simulink model "pd_path_sg"  (R2013b)
settings: Solver=ode45  StartTime=0.0  StopTime=10  RelTol=1e-3
undefined symbols (not defined in the file or in its folder): A, A2, B, C, D, EVAL, i, output_samp_bcoef, PCIN, reg_pk_lim, reg_plim, reg_scale, reg_sr_lim, reg_staclr, reg_txgain, THIS_DATE, W, X, Z
undefined symbols (not defined in the file): lut_address, lut_address_s5, reg_dltap
libraries: xbsIndex_r4 x3819, lut_ram_vhdl x32
(part 5 of 31)

== system pd_path_sg/B_dispatch/vdelay6 ==
  dn : Inport
  x : Inport  Port=2
  ab : Inport  Port=3
  Mux : Mux  Inputs=2
  Reinterpret : xbsIndex_r4/Reinterpret  force_arith_type=on  arith_type="Signed  (2's comp)"  force_bin_pt=on  bin_pt=0  block_type=reinterpret
  Reinterpret1 : xbsIndex_r4/Reinterpret  force_arith_type=on  arith_type="Signed  (2's comp)"  force_bin_pt=on  bin_pt=0  block_type=reinterpret
  Slice : xbsIndex_r4/Slice  nbits=6  boolean_output=off  mode=Lower Bit Location + Width  bit1=0  base1=MSB of Input  bit0=0  base0=LSB of Input  dbl_ovrd=off  block_type=slice
  Slice1 : xbsIndex_r4/Slice  nbits=6  boolean_output=off  mode=Lower Bit Location + Width  bit1=0  base1=MSB of Input  bit0=8  base0=LSB of Input  dbl_ovrd=off  block_type=slice
  Slice2 : xbsIndex_r4/Slice  nbits=16  boolean_output=off  mode=Lower Bit Location + Width  bit1=0  base1=MSB of Input  bit0=16  base0=LSB of Input  dbl_ovrd=off  block_type=slice
  Slice3 : xbsIndex_r4/Slice  nbits=16  boolean_output=off  mode=Lower Bit Location + Width  bit1=0  base1=MSB of Input  bit0=0  base0=LSB of Input  dbl_ovrd=off  block_type=slice
  Slice4 : xbsIndex_r4/Slice  nbits=10  boolean_output=off  mode=Lower Bit Location + Width  bit1=0  base1=MSB of Input  bit0=10  base0=LSB of Input  dbl_ovrd=off  block_type=slice
  Slice5 : xbsIndex_r4/Slice  nbits=10  boolean_output=off  mode=Lower Bit Location + Width  bit1=0  base1=MSB of Input  bit0=0  base0=LSB of Input  dbl_ovrd=off  block_type=slice
  asr0 : xbsIndex_r4/Addressable Shift Register  infer_latency=on  depth=64  initVector=[0]  en=off  use_behavioral_HDL=off  Optimization=Resource  dbl_ovrd=off  block_type=addrsr
      settings: infoedit="Delay of configurable length.  Any element in the delay line can be addressed and driven onto the output port.<br><br>Hardware notes: Generates fast, compact FIFO-style shift registers or delay lines using SRL16/SRL32 mode of the slice LUTs"
  asr1 : xbsIndex_r4/Addressable Shift Register  infer_latency=on  depth=64  initVector=[0]  en=off  use_behavioral_HDL=off  Optimization=Resource  dbl_ovrd=off  block_type=addrsr
      settings: infoedit="Delay of configurable length.  Any element in the delay line can be addressed and driven onto the output port.<br><br>Hardware notes: Generates fast, compact FIFO-style shift registers or delay lines using SRL16/SRL32 mode of the slice LUTs"
  regsp : xbsIndex_r4/Delay  rst=off  infoeditControl=Selection of Reset will increase slice count due to use of real FFs and instead of SRLs  en=off  latency=1  reg_retiming=off  dbl_ovrd=off  block_type=delay
      settings: infoedit=Hardware notes: A delay line is a chain, each link of which is an SRL16 or SRL32 followed by a flip-flop.
  regsp1 : xbsIndex_r4/Delay  rst=off  infoeditControl=Selection of Reset will increase slice count due to use of real FFs and instead of SRLs  en=off  latency=1  reg_retiming=off  dbl_ovrd=off  block_type=delay
      settings: infoedit=Hardware notes: A delay line is a chain, each link of which is an SRL16 or SRL32 followed by a flip-flop.
  y : Outport
  ar : Outport  Port=2
  br : Outport  Port=3
  wires:
  Reinterpret1/1 -> Mux/2
  Reinterpret/1 -> Mux/1
  Mux/1 -> y/1
  Slice3/1 -> Reinterpret1/1
  Slice2/1 -> Reinterpret/1
  dn/1 -> Slice/1, Slice1/1
  Slice5/1 -> br/1
  Slice4/1 -> ar/1
  asr1/1 -> regsp1/1
  asr0/1 -> regsp/1
  x/1 -> asr0/1
  Slice/1 -> asr0/2
  ab/1 -> asr1/1
  Slice1/1 -> asr1/2
  regsp/1 -> Slice2/1, Slice3/1
  regsp1/1 -> Slice5/1, Slice4/1

== system pd_path_sg/B_lut_store/one_lut0 ==
  chn_seq : Inport
  active0 : Inport  Port=2
  active1 : Inport  Port=3
  a : Inport  Port=4
  b : Inport  Port=5
  per_wr : Inport  Port=6
  B : Subsystem
  Bf : Subsystem
  Bp1 : Subsystem
  Bus Selector : BusSelector  OutputSignals=addr,din,we,chnsel,bandsel ,active,per_clk
  Bus Selector1 : BusSelector  OutputSignals=addr,din,we,chnsel,bandsel ,active,per_clk
  Constant : xbsIndex_r4/Constant  const=band_sel  gui_display_data_type=Fixed-point  arith_type=Unsigned  n_bits=1  bin_pt=0  preci_type=Single  exp_width=8  frac_width=24  explicit_period=off  period=1  equ=P=C  opselect=C  inp2=PCIN>>17  opr=+  inp1=P  carry=CIN  dbl_ovrd=off  block_type=constant
  Constant1 : xbsIndex_r4/Constant  const=lut_addr  gui_display_data_type=Fixed-point  arith_type=Unsigned  n_bits=4  bin_pt=0  preci_type=Single  exp_width=8  frac_width=24  explicit_period=off  period=1  equ=P=C  opselect=C  inp2=PCIN>>17  opr=+  inp1=P  carry=CIN  dbl_ovrd=off  block_type=constant
  Constant2 : xbsIndex_r4/Constant  const=0  gui_display_data_type=Fixed-point  arith_type=Unsigned  n_bits=1  bin_pt=0  preci_type=Single  exp_width=8  frac_width=24  explicit_period=off  period=1  equ=P=C  opselect=C  inp2=PCIN>>17  opr=+  inp1=P  carry=CIN  dbl_ovrd=off  block_type=constant
  Constant3 : xbsIndex_r4/Constant  const=band_sel  gui_display_data_type=Fixed-point  arith_type=Unsigned  n_bits=1  bin_pt=0  preci_type=Single  exp_width=8  frac_width=24  explicit_period=off  period=1  equ=P=C  opselect=C  inp2=PCIN>>17  opr=+  inp1=P  carry=CIN  dbl_ovrd=off  block_type=constant
  Constant4 : xbsIndex_r4/Constant  const=lut_addr  gui_display_data_type=Fixed-point  arith_type=Unsigned  n_bits=4  bin_pt=0  preci_type=Single  exp_width=8  frac_width=24  explicit_period=off  period=1  equ=P=C  opselect=C  inp2=PCIN>>17  opr=+  inp1=P  carry=CIN  dbl_ovrd=off  block_type=constant
  Constant5 : xbsIndex_r4/Constant  const=1  gui_display_data_type=Fixed-point  arith_type=Unsigned  n_bits=1  bin_pt=0  preci_type=Single  exp_width=8  frac_width=24  explicit_period=off  period=1  equ=P=C  opselect=C  inp2=PCIN>>17  opr=+  inp1=P  carry=CIN  dbl_ovrd=off  block_type=constant
  Convert : xbsIndex_r4/Convert  gui_display_data_type=Fixed-point  arith_type=Unsigned  n_bits=8  bin_pt=0  float_type=Single  exp_bits=8  fraction_bits=24  quantization=Truncate  overflow=Wrap  en=off  latency=0  pipeline=off  dbl_ovrd=off  block_type=convert
  Delay : xbsIndex_r4/Delay  rst=off  infoeditControl=Selection of Reset will increase slice count due to use of real FFs and instead of SRLs  en=off  latency=4  reg_retiming=off  dbl_ovrd=off  block_type=delay
      settings: infoedit=Hardware notes: A delay line is a chain, each link of which is an SRL16 or SRL32 followed by a flip-flop.
  Delay1 : xbsIndex_r4/Delay  rst=off  infoeditControl=Selection of Reset will increase slice count due to use of real FFs and instead of SRLs  en=off  latency=4  reg_retiming=off  dbl_ovrd=off  block_type=delay
      settings: infoedit=Hardware notes: A delay line is a chain, each link of which is an SRL16 or SRL32 followed by a flip-flop.
  Delay2 : xbsIndex_r4/Delay  rst=off  infoeditControl=Selection of Reset will increase slice count due to use of real FFs and instead of SRLs  en=off  latency=8  reg_retiming=off  dbl_ovrd=off  block_type=delay
      settings: infoedit=Hardware notes: A delay line is a chain, each link of which is an SRL16 or SRL32 followed by a flip-flop.
  Delay{3..6} (4 alike) : xbsIndex_r4/Delay  rst=off  infoeditControl=Selection of Reset will increase slice count due to use of real FFs and instead of SRLs  en=off  latency=1  reg_retiming=off  dbl_ovrd=off  block_type=delay
      settings: infoedit=Hardware notes: A delay line is a chain, each link of which is an SRL16 or SRL32 followed by a flip-flop.
  Reinterpret : xbsIndex_r4/Reinterpret  force_arith_type=on  arith_type="Signed  (2's comp)"  force_bin_pt=on  bin_pt=6  block_type=reinterpret
  addr1 : xbsIndex_r4/Concat  num_inputs=2  dbl_ovrd=off  block_type=concat
  addr3 : xbsIndex_r4/Concat  num_inputs=2  dbl_ovrd=off  block_type=concat
  addr_gen : Subsystem
  interp_a0 : Subsystem
  interp_a1 : Subsystem
  interp_b : Subsystem
  iqslice : Subsystem
  iqslice1 : Subsystem
  iqslice2 : Subsystem
  iqslice3 : Subsystem
  single_ram : lut_ram_vhdl/single_ram
  single_ram1 : lut_ram_vhdl/single_ram
  split_if1 : Subsystem
  split_if2 : Subsystem
  coef_iq : Outport
  wires:
  Convert/1 -> Reinterpret/1
  interp_a1/1(q) -> interp_b/2(b1)
  Delay6/1 -> addr_gen/3(active1)
  Delay5/1 -> addr_gen/2(active0)
  split_if2/2(faddr) -> Convert/1
  Reinterpret/1 -> [Af]
  iqslice/1(ciq) -> interp_a0/1(b0)
  Delay2/1 -> interp_b/3(delta)
  Delay1/1 -> interp_a0/3(delta)
  Delay/1 -> interp_a1/3(delta)
  single_ram/1 -> iqslice/1(d32)
  [A] -> Delay4/1
  [B] -> addr3/1
  [A] -> Delay3/1
  [B_plus] -> addr1/1
  [Bf] -> Delay2/1
  [Af] -> Delay/1
  [Af] -> Delay1/1
  Bf/1(q) -> [Bf]
  B/1(q) -> [B]
  Bp1/1(q) -> [B_plus]
  split_if1/2(faddr) -> Bf/2(delta)
  interp_a0/1(q) -> interp_b/1(b0)
  single_ram1/1 -> iqslice2/1(d32)  "c2"
  single_ram1/2 -> iqslice3/1(d32)  "c3"
  single_ram/2 -> iqslice1/1(d32)  "c1"
  interp_b/1(q) -> coef_iq/1
  b/1 -> split_if1/1(d)
  a/1 -> split_if2/1(d)
  split_if1/1(iaddr) -> B/1(d), Bp1/1(d), Bf/1(iaddr)
  split_if2/1(iaddr) -> [A]
  chn_seq/1 -> addr_gen/1(chn)
  active0/1 -> Delay5/1
  active1/1 -> Delay6/1
  addr1/1 -> addr_gen/4(addr0)
  addr3/1 -> addr_gen/5(addr1)
  addr_gen/1(rd_addr0) -> single_ram/1
  Constant1/1 -> single_ram/2
  Constant/1 -> single_ram/3
  Constant2/1 -> single_ram/4
  per_wr/1 -> Bus Selector1/1, Bus Selector/1
  Bus Selector/7 -> single_ram/11  "<per_clk>"
  Bus Selector/6 -> single_ram/10  "<active>"
  Bus Selector/5 -> single_ram/9  "<bandsel >"
  Bus Selector/4 -> single_ram/8  "<chnsel>"
  Bus Selector/3 -> single_ram/7  "<we>"
  Bus Selector/2 -> single_ram/6  "<din>"
  Bus Selector/1 -> single_ram/5  "<addr>"
  addr_gen/2(rd_addr1) -> single_ram1/1
  Constant3/1 -> single_ram1/3
  Constant4/1 -> single_ram1/2
  Constant5/1 -> single_ram1/4
  Bus Selector1/3 -> single_ram1/7  "<we>"
  Bus Selector1/4 -> single_ram1/8  "<chnsel>"
  Bus Selector1/5 -> single_ram1/9  "<bandsel >"
  Bus Selector1/1 -> single_ram1/5  "<addr>"
  Bus Selector1/7 -> single_ram1/11  "<per_clk>"
  Bus Selector1/2 -> single_ram1/6  "<din>"
  Bus Selector1/6 -> single_ram1/10  "<active>"
  Delay3/1 -> addr1/2
  Delay4/1 -> addr3/2
  iqslice1/1(ciq) -> interp_a0/2(b1)
  iqslice2/1(ciq) -> interp_a1/1(b0)
  iqslice3/1(ciq) -> interp_a1/2(b1)

== system pd_path_sg/B_lut_store/one_lut1 ==
  chn_seq : Inport
  active0 : Inport  Port=2
  active1 : Inport  Port=3
  a : Inport  Port=4
  b : Inport  Port=5
  per_wr : Inport  Port=6
  B : Subsystem
  Bf : Subsystem
  Bp1 : Subsystem
  Bus Selector : BusSelector  OutputSignals=addr,din,we,chnsel,bandsel ,active,per_clk
  Bus Selector1 : BusSelector  OutputSignals=addr,din,we,chnsel,bandsel ,active,per_clk
  Constant : xbsIndex_r4/Constant  const=band_sel  gui_display_data_type=Fixed-point  arith_type=Unsigned  n_bits=1  bin_pt=0  preci_type=Single  exp_width=8  frac_width=24  explicit_period=off  period=1  equ=P=C  opselect=C  inp2=PCIN>>17  opr=+  inp1=P  carry=CIN  dbl_ovrd=off  block_type=constant
  Constant1 : xbsIndex_r4/Constant  const=lut_addr  gui_display_data_type=Fixed-point  arith_type=Unsigned  n_bits=4  bin_pt=0  preci_type=Single  exp_width=8  frac_width=24  explicit_period=off  period=1  equ=P=C  opselect=C  inp2=PCIN>>17  opr=+  inp1=P  carry=CIN  dbl_ovrd=off  block_type=constant
  Constant2 : xbsIndex_r4/Constant  const=0  gui_display_data_type=Fixed-point  arith_type=Unsigned  n_bits=1  bin_pt=0  preci_type=Single  exp_width=8  frac_width=24  explicit_period=off  period=1  equ=P=C  opselect=C  inp2=PCIN>>17  opr=+  inp1=P  carry=CIN  dbl_ovrd=off  block_type=constant
  Constant3 : xbsIndex_r4/Constant  const=band_sel  gui_display_data_type=Fixed-point  arith_type=Unsigned  n_bits=1  bin_pt=0  preci_type=Single  exp_width=8  frac_width=24  explicit_period=off  period=1  equ=P=C  opselect=C  inp2=PCIN>>17  opr=+  inp1=P  carry=CIN  dbl_ovrd=off  block_type=constant
  Constant4 : xbsIndex_r4/Constant  const=lut_addr  gui_display_data_type=Fixed-point  arith_type=Unsigned  n_bits=4  bin_pt=0  preci_type=Single  exp_width=8  frac_width=24  explicit_period=off  period=1  equ=P=C  opselect=C  inp2=PCIN>>17  opr=+  inp1=P  carry=CIN  dbl_ovrd=off  block_type=constant
  Constant5 : xbsIndex_r4/Constant  const=1  gui_display_data_type=Fixed-point  arith_type=Unsigned  n_bits=1  bin_pt=0  preci_type=Single  exp_width=8  frac_width=24  explicit_period=off  period=1  equ=P=C  opselect=C  inp2=PCIN>>17  opr=+  inp1=P  carry=CIN  dbl_ovrd=off  block_type=constant
  Convert : xbsIndex_r4/Convert  gui_display_data_type=Fixed-point  arith_type=Unsigned  n_bits=8  bin_pt=0  float_type=Single  exp_bits=8  fraction_bits=24  quantization=Truncate  overflow=Wrap  en=off  latency=0  pipeline=off  dbl_ovrd=off  block_type=convert
  Delay : xbsIndex_r4/Delay  rst=off  infoeditControl=Selection of Reset will increase slice count due to use of real FFs and instead of SRLs  en=off  latency=4  reg_retiming=off  dbl_ovrd=off  block_type=delay
      settings: infoedit=Hardware notes: A delay line is a chain, each link of which is an SRL16 or SRL32 followed by a flip-flop.
  Delay1 : xbsIndex_r4/Delay  rst=off  infoeditControl=Selection of Reset will increase slice count due to use of real FFs and instead of SRLs  en=off  latency=4  reg_retiming=off  dbl_ovrd=off  block_type=delay
      settings: infoedit=Hardware notes: A delay line is a chain, each link of which is an SRL16 or SRL32 followed by a flip-flop.
  Delay2 : xbsIndex_r4/Delay  rst=off  infoeditControl=Selection of Reset will increase slice count due to use of real FFs and instead of SRLs  en=off  latency=8  reg_retiming=off  dbl_ovrd=off  block_type=delay
      settings: infoedit=Hardware notes: A delay line is a chain, each link of which is an SRL16 or SRL32 followed by a flip-flop.
  Delay{3..6} (4 alike) : xbsIndex_r4/Delay  rst=off  infoeditControl=Selection of Reset will increase slice count due to use of real FFs and instead of SRLs  en=off  latency=1  reg_retiming=off  dbl_ovrd=off  block_type=delay
      settings: infoedit=Hardware notes: A delay line is a chain, each link of which is an SRL16 or SRL32 followed by a flip-flop.
  Reinterpret : xbsIndex_r4/Reinterpret  force_arith_type=on  arith_type="Signed  (2's comp)"  force_bin_pt=on  bin_pt=6  block_type=reinterpret
  addr1 : xbsIndex_r4/Concat  num_inputs=2  dbl_ovrd=off  block_type=concat
  addr3 : xbsIndex_r4/Concat  num_inputs=2  dbl_ovrd=off  block_type=concat
  addr_gen : Subsystem
  interp_a0 : Subsystem
  interp_a1 : Subsystem
  interp_b : Subsystem
  iqslice : Subsystem
  iqslice1 : Subsystem
  iqslice2 : Subsystem
  iqslice3 : Subsystem
  single_ram : lut_ram_vhdl/single_ram
  single_ram1 : lut_ram_vhdl/single_ram
  split_if1 : Subsystem
  split_if2 : Subsystem
  coef_iq : Outport
  wires:
  iqslice3/1(ciq) -> interp_a1/2(b1)
  iqslice2/1(ciq) -> interp_a1/1(b0)
  iqslice1/1(ciq) -> interp_a0/2(b1)
  Delay4/1 -> addr3/2
  Delay3/1 -> addr1/2
  Bus Selector1/6 -> single_ram1/10  "<active>"
  Bus Selector1/2 -> single_ram1/6  "<din>"
  Bus Selector1/7 -> single_ram1/11  "<per_clk>"
  Bus Selector1/1 -> single_ram1/5  "<addr>"
  Bus Selector1/5 -> single_ram1/9  "<bandsel >"
  Bus Selector1/4 -> single_ram1/8  "<chnsel>"
  Bus Selector1/3 -> single_ram1/7  "<we>"
  Constant5/1 -> single_ram1/4
  Constant4/1 -> single_ram1/2
  Constant3/1 -> single_ram1/3
  addr_gen/2(rd_addr1) -> single_ram1/1
  Bus Selector/1 -> single_ram/5  "<addr>"
  Bus Selector/2 -> single_ram/6  "<din>"
  Bus Selector/3 -> single_ram/7  "<we>"
  Bus Selector/4 -> single_ram/8  "<chnsel>"
  Bus Selector/5 -> single_ram/9  "<bandsel >"
  Bus Selector/6 -> single_ram/10  "<active>"
  Bus Selector/7 -> single_ram/11  "<per_clk>"
  per_wr/1 -> Bus Selector/1, Bus Selector1/1
  Constant2/1 -> single_ram/4
  Constant/1 -> single_ram/3
  Constant1/1 -> single_ram/2
  addr_gen/1(rd_addr0) -> single_ram/1
  addr3/1 -> addr_gen/5(addr1)
  addr1/1 -> addr_gen/4(addr0)
  active1/1 -> Delay6/1
  active0/1 -> Delay5/1
  chn_seq/1 -> addr_gen/1(chn)
  split_if2/1(iaddr) -> [A]
  split_if1/1(iaddr) -> Bf/1(iaddr), Bp1/1(d), B/1(d)
  a/1 -> split_if2/1(d)
  b/1 -> split_if1/1(d)
  interp_b/1(q) -> coef_iq/1
  single_ram/2 -> iqslice1/1(d32)  "c1"
  single_ram1/2 -> iqslice3/1(d32)  "c3"
  single_ram1/1 -> iqslice2/1(d32)  "c2"
  interp_a0/1(q) -> interp_b/1(b0)
  split_if1/2(faddr) -> Bf/2(delta)
  Bp1/1(q) -> [B_plus]
  B/1(q) -> [B]
  Bf/1(q) -> [Bf]
  [Af] -> Delay1/1
  [Af] -> Delay/1
  [Bf] -> Delay2/1
  [B_plus] -> addr1/1
  [A] -> Delay3/1
  [B] -> addr3/1
  [A] -> Delay4/1
  single_ram/1 -> iqslice/1(d32)
  Delay/1 -> interp_a1/3(delta)
  Delay1/1 -> interp_a0/3(delta)
  Delay2/1 -> interp_b/3(delta)
  iqslice/1(ciq) -> interp_a0/1(b0)
  Reinterpret/1 -> [Af]
  split_if2/2(faddr) -> Convert/1
  Delay5/1 -> addr_gen/2(active0)
  Delay6/1 -> addr_gen/3(active1)
  interp_a1/1(q) -> interp_b/2(b1)
  Convert/1 -> Reinterpret/1

== system pd_path_sg/B_lut_store/one_lut2 ==
  chn_seq : Inport
  active0 : Inport  Port=2
  active1 : Inport  Port=3
  a : Inport  Port=4
  b : Inport  Port=5
  per_wr : Inport  Port=6
  B : Subsystem
  Bf : Subsystem
  Bp1 : Subsystem
  Bus Selector : BusSelector  OutputSignals=addr,din,we,chnsel,bandsel ,active,per_clk
  Bus Selector1 : BusSelector  OutputSignals=addr,din,we,chnsel,bandsel ,active,per_clk
  Constant : xbsIndex_r4/Constant  const=band_sel  gui_display_data_type=Fixed-point  arith_type=Unsigned  n_bits=1  bin_pt=0  preci_type=Single  exp_width=8  frac_width=24  explicit_period=off  period=1  equ=P=C  opselect=C  inp2=PCIN>>17  opr=+  inp1=P  carry=CIN  dbl_ovrd=off  block_type=constant
  Constant1 : xbsIndex_r4/Constant  const=lut_addr  gui_display_data_type=Fixed-point  arith_type=Unsigned  n_bits=4  bin_pt=0  preci_type=Single  exp_width=8  frac_width=24  explicit_period=off  period=1  equ=P=C  opselect=C  inp2=PCIN>>17  opr=+  inp1=P  carry=CIN  dbl_ovrd=off  block_type=constant
  Constant2 : xbsIndex_r4/Constant  const=0  gui_display_data_type=Fixed-point  arith_type=Unsigned  n_bits=1  bin_pt=0  preci_type=Single  exp_width=8  frac_width=24  explicit_period=off  period=1  equ=P=C  opselect=C  inp2=PCIN>>17  opr=+  inp1=P  carry=CIN  dbl_ovrd=off  block_type=constant
  Constant3 : xbsIndex_r4/Constant  const=band_sel  gui_display_data_type=Fixed-point  arith_type=Unsigned  n_bits=1  bin_pt=0  preci_type=Single  exp_width=8  frac_width=24  explicit_period=off  period=1  equ=P=C  opselect=C  inp2=PCIN>>17  opr=+  inp1=P  carry=CIN  dbl_ovrd=off  block_type=constant
  Constant4 : xbsIndex_r4/Constant  const=lut_addr  gui_display_data_type=Fixed-point  arith_type=Unsigned  n_bits=4  bin_pt=0  preci_type=Single  exp_width=8  frac_width=24  explicit_period=off  period=1  equ=P=C  opselect=C  inp2=PCIN>>17  opr=+  inp1=P  carry=CIN  dbl_ovrd=off  block_type=constant
  Constant5 : xbsIndex_r4/Constant  const=1  gui_display_data_type=Fixed-point  arith_type=Unsigned  n_bits=1  bin_pt=0  preci_type=Single  exp_width=8  frac_width=24  explicit_period=off  period=1  equ=P=C  opselect=C  inp2=PCIN>>17  opr=+  inp1=P  carry=CIN  dbl_ovrd=off  block_type=constant
  Convert : xbsIndex_r4/Convert  gui_display_data_type=Fixed-point  arith_type=Unsigned  n_bits=8  bin_pt=0  float_type=Single  exp_bits=8  fraction_bits=24  quantization=Truncate  overflow=Wrap  en=off  latency=0  pipeline=off  dbl_ovrd=off  block_type=convert
  Delay : xbsIndex_r4/Delay  rst=off  infoeditControl=Selection of Reset will increase slice count due to use of real FFs and instead of SRLs  en=off  latency=4  reg_retiming=off  dbl_ovrd=off  block_type=delay
      settings: infoedit=Hardware notes: A delay line is a chain, each link of which is an SRL16 or SRL32 followed by a flip-flop.
  Delay1 : xbsIndex_r4/Delay  rst=off  infoeditControl=Selection of Reset will increase slice count due to use of real FFs and instead of SRLs  en=off  latency=4  reg_retiming=off  dbl_ovrd=off  block_type=delay
      settings: infoedit=Hardware notes: A delay line is a chain, each link of which is an SRL16 or SRL32 followed by a flip-flop.
  Delay2 : xbsIndex_r4/Delay  rst=off  infoeditControl=Selection of Reset will increase slice count due to use of real FFs and instead of SRLs  en=off  latency=8  reg_retiming=off  dbl_ovrd=off  block_type=delay
      settings: infoedit=Hardware notes: A delay line is a chain, each link of which is an SRL16 or SRL32 followed by a flip-flop.
  Delay{3..6} (4 alike) : xbsIndex_r4/Delay  rst=off  infoeditControl=Selection of Reset will increase slice count due to use of real FFs and instead of SRLs  en=off  latency=1  reg_retiming=off  dbl_ovrd=off  block_type=delay
      settings: infoedit=Hardware notes: A delay line is a chain, each link of which is an SRL16 or SRL32 followed by a flip-flop.
  Reinterpret : xbsIndex_r4/Reinterpret  force_arith_type=on  arith_type="Signed  (2's comp)"  force_bin_pt=on  bin_pt=6  block_type=reinterpret
  addr1 : xbsIndex_r4/Concat  num_inputs=2  dbl_ovrd=off  block_type=concat
  addr3 : xbsIndex_r4/Concat  num_inputs=2  dbl_ovrd=off  block_type=concat
  addr_gen : Subsystem
  interp_a0 : Subsystem
  interp_a1 : Subsystem
  interp_b : Subsystem
  iqslice : Subsystem
  iqslice1 : Subsystem
  iqslice2 : Subsystem
  iqslice3 : Subsystem
  single_ram : lut_ram_vhdl/single_ram
  single_ram1 : lut_ram_vhdl/single_ram
  split_if1 : Subsystem
  split_if2 : Subsystem
  coef_iq : Outport
  wires:
  Convert/1 -> Reinterpret/1
  interp_a1/1(q) -> interp_b/2(b1)
  Delay6/1 -> addr_gen/3(active1)
  Delay5/1 -> addr_gen/2(active0)
  split_if2/2(faddr) -> Convert/1
  Reinterpret/1 -> [Af]
  iqslice/1(ciq) -> interp_a0/1(b0)
  Delay2/1 -> interp_b/3(delta)
  Delay1/1 -> interp_a0/3(delta)
  Delay/1 -> interp_a1/3(delta)
  single_ram/1 -> iqslice/1(d32)
  [A] -> Delay4/1
  [B] -> addr3/1
  [A] -> Delay3/1
  [B_plus] -> addr1/1
  [Bf] -> Delay2/1
  [Af] -> Delay/1
  [Af] -> Delay1/1
  Bf/1(q) -> [Bf]
  B/1(q) -> [B]
  Bp1/1(q) -> [B_plus]
  split_if1/2(faddr) -> Bf/2(delta)
  interp_a0/1(q) -> interp_b/1(b0)
  single_ram1/1 -> iqslice2/1(d32)  "c2"
  single_ram1/2 -> iqslice3/1(d32)  "c3"
  single_ram/2 -> iqslice1/1(d32)  "c1"
  interp_b/1(q) -> coef_iq/1
  b/1 -> split_if1/1(d)
  a/1 -> split_if2/1(d)
  split_if1/1(iaddr) -> B/1(d), Bp1/1(d), Bf/1(iaddr)
  split_if2/1(iaddr) -> [A]
  chn_seq/1 -> addr_gen/1(chn)
  active0/1 -> Delay5/1
  active1/1 -> Delay6/1
  addr1/1 -> addr_gen/4(addr0)
  addr3/1 -> addr_gen/5(addr1)
  addr_gen/1(rd_addr0) -> single_ram/1
  Constant1/1 -> single_ram/2
  Constant/1 -> single_ram/3
  Constant2/1 -> single_ram/4
  per_wr/1 -> Bus Selector1/1, Bus Selector/1
  Bus Selector/7 -> single_ram/11  "<per_clk>"
  Bus Selector/6 -> single_ram/10  "<active>"
  Bus Selector/5 -> single_ram/9  "<bandsel >"
  Bus Selector/4 -> single_ram/8  "<chnsel>"
  Bus Selector/3 -> single_ram/7  "<we>"
  Bus Selector/2 -> single_ram/6  "<din>"
  Bus Selector/1 -> single_ram/5  "<addr>"
  addr_gen/2(rd_addr1) -> single_ram1/1
  Constant3/1 -> single_ram1/3
  Constant4/1 -> single_ram1/2
  Constant5/1 -> single_ram1/4
  Bus Selector1/3 -> single_ram1/7  "<we>"
  Bus Selector1/4 -> single_ram1/8  "<chnsel>"
  Bus Selector1/5 -> single_ram1/9  "<bandsel >"
  Bus Selector1/1 -> single_ram1/5  "<addr>"
  Bus Selector1/7 -> single_ram1/11  "<per_clk>"
  Bus Selector1/2 -> single_ram1/6  "<din>"
  Bus Selector1/6 -> single_ram1/10  "<active>"
  Delay3/1 -> addr1/2
  Delay4/1 -> addr3/2
  iqslice1/1(ciq) -> interp_a0/2(b1)
  iqslice2/1(ciq) -> interp_a1/1(b0)
  iqslice3/1(ciq) -> interp_a1/2(b1)

== system pd_path_sg/B_lut_store/one_lut3 ==
  chn_seq : Inport
  active0 : Inport  Port=2
  active1 : Inport  Port=3
  a : Inport  Port=4
  b : Inport  Port=5
  per_wr : Inport  Port=6
  B : Subsystem
  Bf : Subsystem
  Bp1 : Subsystem
  Bus Selector : BusSelector  OutputSignals=addr,din,we,chnsel,bandsel ,active,per_clk
  Bus Selector1 : BusSelector  OutputSignals=addr,din,we,chnsel,bandsel ,active,per_clk
  Constant : xbsIndex_r4/Constant  const=band_sel  gui_display_data_type=Fixed-point  arith_type=Unsigned  n_bits=1  bin_pt=0  preci_type=Single  exp_width=8  frac_width=24  explicit_period=off  period=1  equ=P=C  opselect=C  inp2=PCIN>>17  opr=+  inp1=P  carry=CIN  dbl_ovrd=off  block_type=constant
  Constant1 : xbsIndex_r4/Constant  const=lut_addr  gui_display_data_type=Fixed-point  arith_type=Unsigned  n_bits=4  bin_pt=0  preci_type=Single  exp_width=8  frac_width=24  explicit_period=off  period=1  equ=P=C  opselect=C  inp2=PCIN>>17  opr=+  inp1=P  carry=CIN  dbl_ovrd=off  block_type=constant
  Constant2 : xbsIndex_r4/Constant  const=0  gui_display_data_type=Fixed-point  arith_type=Unsigned  n_bits=1  bin_pt=0  preci_type=Single  exp_width=8  frac_width=24  explicit_period=off  period=1  equ=P=C  opselect=C  inp2=PCIN>>17  opr=+  inp1=P  carry=CIN  dbl_ovrd=off  block_type=constant
  Constant3 : xbsIndex_r4/Constant  const=band_sel  gui_display_data_type=Fixed-point  arith_type=Unsigned  n_bits=1  bin_pt=0  preci_type=Single  exp_width=8  frac_width=24  explicit_period=off  period=1  equ=P=C  opselect=C  inp2=PCIN>>17  opr=+  inp1=P  carry=CIN  dbl_ovrd=off  block_type=constant
  Constant4 : xbsIndex_r4/Constant  const=lut_addr  gui_display_data_type=Fixed-point  arith_type=Unsigned  n_bits=4  bin_pt=0  preci_type=Single  exp_width=8  frac_width=24  explicit_period=off  period=1  equ=P=C  opselect=C  inp2=PCIN>>17  opr=+  inp1=P  carry=CIN  dbl_ovrd=off  block_type=constant
  Constant5 : xbsIndex_r4/Constant  const=1  gui_display_data_type=Fixed-point  arith_type=Unsigned  n_bits=1  bin_pt=0  preci_type=Single  exp_width=8  frac_width=24  explicit_period=off  period=1  equ=P=C  opselect=C  inp2=PCIN>>17  opr=+  inp1=P  carry=CIN  dbl_ovrd=off  block_type=constant
  Convert : xbsIndex_r4/Convert  gui_display_data_type=Fixed-point  arith_type=Unsigned  n_bits=8  bin_pt=0  float_type=Single  exp_bits=8  fraction_bits=24  quantization=Truncate  overflow=Wrap  en=off  latency=0  pipeline=off  dbl_ovrd=off  block_type=convert
  Delay : xbsIndex_r4/Delay  rst=off  infoeditControl=Selection of Reset will increase slice count due to use of real FFs and instead of SRLs  en=off  latency=4  reg_retiming=off  dbl_ovrd=off  block_type=delay
      settings: infoedit=Hardware notes: A delay line is a chain, each link of which is an SRL16 or SRL32 followed by a flip-flop.
  Delay1 : xbsIndex_r4/Delay  rst=off  infoeditControl=Selection of Reset will increase slice count due to use of real FFs and instead of SRLs  en=off  latency=4  reg_retiming=off  dbl_ovrd=off  block_type=delay
      settings: infoedit=Hardware notes: A delay line is a chain, each link of which is an SRL16 or SRL32 followed by a flip-flop.
  Delay2 : xbsIndex_r4/Delay  rst=off  infoeditControl=Selection of Reset will increase slice count due to use of real FFs and instead of SRLs  en=off  latency=8  reg_retiming=off  dbl_ovrd=off  block_type=delay
      settings: infoedit=Hardware notes: A delay line is a chain, each link of which is an SRL16 or SRL32 followed by a flip-flop.
  Delay{3..6} (4 alike) : xbsIndex_r4/Delay  rst=off  infoeditControl=Selection of Reset will increase slice count due to use of real FFs and instead of SRLs  en=off  latency=1  reg_retiming=off  dbl_ovrd=off  block_type=delay
      settings: infoedit=Hardware notes: A delay line is a chain, each link of which is an SRL16 or SRL32 followed by a flip-flop.
  Reinterpret : xbsIndex_r4/Reinterpret  force_arith_type=on  arith_type="Signed  (2's comp)"  force_bin_pt=on  bin_pt=6  block_type=reinterpret
  addr1 : xbsIndex_r4/Concat  num_inputs=2  dbl_ovrd=off  block_type=concat
  addr3 : xbsIndex_r4/Concat  num_inputs=2  dbl_ovrd=off  block_type=concat
  addr_gen : Subsystem
  interp_a0 : Subsystem
  interp_a1 : Subsystem
  interp_b : Subsystem
  iqslice : Subsystem
  iqslice1 : Subsystem
  iqslice2 : Subsystem
  iqslice3 : Subsystem
  single_ram : lut_ram_vhdl/single_ram
  single_ram1 : lut_ram_vhdl/single_ram
  split_if1 : Subsystem
  split_if2 : Subsystem
  coef_iq : Outport
  wires:
  iqslice3/1(ciq) -> interp_a1/2(b1)
  iqslice2/1(ciq) -> interp_a1/1(b0)
  iqslice1/1(ciq) -> interp_a0/2(b1)
  Delay4/1 -> addr3/2
  Delay3/1 -> addr1/2
  Bus Selector1/6 -> single_ram1/10  "<active>"
  Bus Selector1/2 -> single_ram1/6  "<din>"
  Bus Selector1/7 -> single_ram1/11  "<per_clk>"
  Bus Selector1/1 -> single_ram1/5  "<addr>"
  Bus Selector1/5 -> single_ram1/9  "<bandsel >"
  Bus Selector1/4 -> single_ram1/8  "<chnsel>"
  Bus Selector1/3 -> single_ram1/7  "<we>"
  Constant5/1 -> single_ram1/4
  Constant4/1 -> single_ram1/2
  Constant3/1 -> single_ram1/3
  addr_gen/2(rd_addr1) -> single_ram1/1
  Bus Selector/1 -> single_ram/5  "<addr>"
  Bus Selector/2 -> single_ram/6  "<din>"
  Bus Selector/3 -> single_ram/7  "<we>"
  Bus Selector/4 -> single_ram/8  "<chnsel>"
  Bus Selector/5 -> single_ram/9  "<bandsel >"
  Bus Selector/6 -> single_ram/10  "<active>"
  Bus Selector/7 -> single_ram/11  "<per_clk>"
  per_wr/1 -> Bus Selector/1, Bus Selector1/1
  Constant2/1 -> single_ram/4
  Constant/1 -> single_ram/3
  Constant1/1 -> single_ram/2
  addr_gen/1(rd_addr0) -> single_ram/1
  addr3/1 -> addr_gen/5(addr1)
  addr1/1 -> addr_gen/4(addr0)
  active1/1 -> Delay6/1
  active0/1 -> Delay5/1
  chn_seq/1 -> addr_gen/1(chn)
  split_if2/1(iaddr) -> [A]
  split_if1/1(iaddr) -> Bf/1(iaddr), Bp1/1(d), B/1(d)
  a/1 -> split_if2/1(d)
  b/1 -> split_if1/1(d)
  interp_b/1(q) -> coef_iq/1
  single_ram/2 -> iqslice1/1(d32)  "c1"
  single_ram1/2 -> iqslice3/1(d32)  "c3"
  single_ram1/1 -> iqslice2/1(d32)  "c2"
  interp_a0/1(q) -> interp_b/1(b0)
  split_if1/2(faddr) -> Bf/2(delta)
  Bp1/1(q) -> [B_plus]
  B/1(q) -> [B]
  Bf/1(q) -> [Bf]
  [Af] -> Delay1/1
  [Af] -> Delay/1
  [Bf] -> Delay2/1
  [B_plus] -> addr1/1
  [A] -> Delay3/1
  [B] -> addr3/1
  [A] -> Delay4/1
  single_ram/1 -> iqslice/1(d32)
  Delay/1 -> interp_a1/3(delta)
  Delay1/1 -> interp_a0/3(delta)
  Delay2/1 -> interp_b/3(delta)
  iqslice/1(ciq) -> interp_a0/1(b0)
  Reinterpret/1 -> [Af]
  split_if2/2(faddr) -> Convert/1
  Delay5/1 -> addr_gen/2(active0)
  Delay6/1 -> addr_gen/3(active1)
  interp_a1/1(q) -> interp_b/2(b1)
  Convert/1 -> Reinterpret/1

== system pd_path_sg/B_lut_store/one_lut4 ==
  chn_seq : Inport
  active0 : Inport  Port=2
  active1 : Inport  Port=3
  a : Inport  Port=4
  b : Inport  Port=5
  per_wr : Inport  Port=6
  B : Subsystem
  Bf : Subsystem
  Bp1 : Subsystem
  Bus Selector : BusSelector  OutputSignals=addr,din,we,chnsel,bandsel ,active,per_clk
  Bus Selector1 : BusSelector  OutputSignals=addr,din,we,chnsel,bandsel ,active,per_clk
  Constant : xbsIndex_r4/Constant  const=band_sel  gui_display_data_type=Fixed-point  arith_type=Unsigned  n_bits=1  bin_pt=0  preci_type=Single  exp_width=8  frac_width=24  explicit_period=off  period=1  equ=P=C  opselect=C  inp2=PCIN>>17  opr=+  inp1=P  carry=CIN  dbl_ovrd=off  block_type=constant
  Constant1 : xbsIndex_r4/Constant  const=lut_addr  gui_display_data_type=Fixed-point  arith_type=Unsigned  n_bits=4  bin_pt=0  preci_type=Single  exp_width=8  frac_width=24  explicit_period=off  period=1  equ=P=C  opselect=C  inp2=PCIN>>17  opr=+  inp1=P  carry=CIN  dbl_ovrd=off  block_type=constant
  Constant2 : xbsIndex_r4/Constant  const=0  gui_display_data_type=Fixed-point  arith_type=Unsigned  n_bits=1  bin_pt=0  preci_type=Single  exp_width=8  frac_width=24  explicit_period=off  period=1  equ=P=C  opselect=C  inp2=PCIN>>17  opr=+  inp1=P  carry=CIN  dbl_ovrd=off  block_type=constant
  Constant3 : xbsIndex_r4/Constant  const=band_sel  gui_display_data_type=Fixed-point  arith_type=Unsigned  n_bits=1  bin_pt=0  preci_type=Single  exp_width=8  frac_width=24  explicit_period=off  period=1  equ=P=C  opselect=C  inp2=PCIN>>17  opr=+  inp1=P  carry=CIN  dbl_ovrd=off  block_type=constant
  Constant4 : xbsIndex_r4/Constant  const=lut_addr  gui_display_data_type=Fixed-point  arith_type=Unsigned  n_bits=4  bin_pt=0  preci_type=Single  exp_width=8  frac_width=24  explicit_period=off  period=1  equ=P=C  opselect=C  inp2=PCIN>>17  opr=+  inp1=P  carry=CIN  dbl_ovrd=off  block_type=constant
  Constant5 : xbsIndex_r4/Constant  const=1  gui_display_data_type=Fixed-point  arith_type=Unsigned  n_bits=1  bin_pt=0  preci_type=Single  exp_width=8  frac_width=24  explicit_period=off  period=1  equ=P=C  opselect=C  inp2=PCIN>>17  opr=+  inp1=P  carry=CIN  dbl_ovrd=off  block_type=constant
  Convert : xbsIndex_r4/Convert  gui_display_data_type=Fixed-point  arith_type=Unsigned  n_bits=8  bin_pt=0  float_type=Single  exp_bits=8  fraction_bits=24  quantization=Truncate  overflow=Wrap  en=off  latency=0  pipeline=off  dbl_ovrd=off  block_type=convert
  Delay : xbsIndex_r4/Delay  rst=off  infoeditControl=Selection of Reset will increase slice count due to use of real FFs and instead of SRLs  en=off  latency=4  reg_retiming=off  dbl_ovrd=off  block_type=delay
      settings: infoedit=Hardware notes: A delay line is a chain, each link of which is an SRL16 or SRL32 followed by a flip-flop.
  Delay1 : xbsIndex_r4/Delay  rst=off  infoeditControl=Selection of Reset will increase slice count due to use of real FFs and instead of SRLs  en=off  latency=4  reg_retiming=off  dbl_ovrd=off  block_type=delay
      settings: infoedit=Hardware notes: A delay line is a chain, each link of which is an SRL16 or SRL32 followed by a flip-flop.
  Delay2 : xbsIndex_r4/Delay  rst=off  infoeditControl=Selection of Reset will increase slice count due to use of real FFs and instead of SRLs  en=off  latency=8  reg_retiming=off  dbl_ovrd=off  block_type=delay
      settings: infoedit=Hardware notes: A delay line is a chain, each link of which is an SRL16 or SRL32 followed by a flip-flop.
  Delay{3..6} (4 alike) : xbsIndex_r4/Delay  rst=off  infoeditControl=Selection of Reset will increase slice count due to use of real FFs and instead of SRLs  en=off  latency=1  reg_retiming=off  dbl_ovrd=off  block_type=delay
      settings: infoedit=Hardware notes: A delay line is a chain, each link of which is an SRL16 or SRL32 followed by a flip-flop.
  Reinterpret : xbsIndex_r4/Reinterpret  force_arith_type=on  arith_type="Signed  (2's comp)"  force_bin_pt=on  bin_pt=6  block_type=reinterpret
  addr1 : xbsIndex_r4/Concat  num_inputs=2  dbl_ovrd=off  block_type=concat
  addr3 : xbsIndex_r4/Concat  num_inputs=2  dbl_ovrd=off  block_type=concat
  addr_gen : Subsystem
  interp_a0 : Subsystem
  interp_a1 : Subsystem
  interp_b : Subsystem
  iqslice : Subsystem
  iqslice1 : Subsystem
  iqslice2 : Subsystem
  iqslice3 : Subsystem
  single_ram : lut_ram_vhdl/single_ram
  single_ram1 : lut_ram_vhdl/single_ram
  split_if1 : Subsystem
  split_if2 : Subsystem
  coef_iq : Outport
  wires:
  Convert/1 -> Reinterpret/1
  interp_a1/1(q) -> interp_b/2(b1)
  Delay6/1 -> addr_gen/3(active1)
  Delay5/1 -> addr_gen/2(active0)
  split_if2/2(faddr) -> Convert/1
  Reinterpret/1 -> [Af]
  iqslice/1(ciq) -> interp_a0/1(b0)
  Delay2/1 -> interp_b/3(delta)
  Delay1/1 -> interp_a0/3(delta)
  Delay/1 -> interp_a1/3(delta)
  single_ram/1 -> iqslice/1(d32)
  [A] -> Delay4/1
  [B] -> addr3/1
  [A] -> Delay3/1
  [B_plus] -> addr1/1
  [Bf] -> Delay2/1
  [Af] -> Delay/1
  [Af] -> Delay1/1
  Bf/1(q) -> [Bf]
  B/1(q) -> [B]
  Bp1/1(q) -> [B_plus]
  split_if1/2(faddr) -> Bf/2(delta)
  interp_a0/1(q) -> interp_b/1(b0)
  single_ram1/1 -> iqslice2/1(d32)  "c2"
  single_ram1/2 -> iqslice3/1(d32)  "c3"
  single_ram/2 -> iqslice1/1(d32)  "c1"
  interp_b/1(q) -> coef_iq/1
  b/1 -> split_if1/1(d)
  a/1 -> split_if2/1(d)
  split_if1/1(iaddr) -> B/1(d), Bp1/1(d), Bf/1(iaddr)
  split_if2/1(iaddr) -> [A]
  chn_seq/1 -> addr_gen/1(chn)
  active0/1 -> Delay5/1
  active1/1 -> Delay6/1
  addr1/1 -> addr_gen/4(addr0)
  addr3/1 -> addr_gen/5(addr1)
  addr_gen/1(rd_addr0) -> single_ram/1
  Constant1/1 -> single_ram/2
  Constant/1 -> single_ram/3
  Constant2/1 -> single_ram/4
  per_wr/1 -> Bus Selector1/1, Bus Selector/1
  Bus Selector/7 -> single_ram/11  "<per_clk>"
  Bus Selector/6 -> single_ram/10  "<active>"
  Bus Selector/5 -> single_ram/9  "<bandsel >"
  Bus Selector/4 -> single_ram/8  "<chnsel>"
  Bus Selector/3 -> single_ram/7  "<we>"
  Bus Selector/2 -> single_ram/6  "<din>"
  Bus Selector/1 -> single_ram/5  "<addr>"
  addr_gen/2(rd_addr1) -> single_ram1/1
  Constant3/1 -> single_ram1/3
  Constant4/1 -> single_ram1/2
  Constant5/1 -> single_ram1/4
  Bus Selector1/3 -> single_ram1/7  "<we>"
  Bus Selector1/4 -> single_ram1/8  "<chnsel>"
  Bus Selector1/5 -> single_ram1/9  "<bandsel >"
  Bus Selector1/1 -> single_ram1/5  "<addr>"
  Bus Selector1/7 -> single_ram1/11  "<per_clk>"
  Bus Selector1/2 -> single_ram1/6  "<din>"
  Bus Selector1/6 -> single_ram1/10  "<active>"
  Delay3/1 -> addr1/2
  Delay4/1 -> addr3/2
  iqslice1/1(ciq) -> interp_a0/2(b1)
  iqslice2/1(ciq) -> interp_a1/1(b0)
  iqslice3/1(ciq) -> interp_a1/2(b1)

== system pd_path_sg/B_lut_store/one_lut5 ==
  chn_seq : Inport
  active0 : Inport  Port=2
  active1 : Inport  Port=3
  a : Inport  Port=4
  b : Inport  Port=5
  per_wr : Inport  Port=6
  B : Subsystem
  Bf : Subsystem
  Bp1 : Subsystem
  Bus Selector : BusSelector  OutputSignals=addr,din,we,chnsel,bandsel ,active,per_clk
  Bus Selector1 : BusSelector  OutputSignals=addr,din,we,chnsel,bandsel ,active,per_clk
  Constant : xbsIndex_r4/Constant  const=band_sel  gui_display_data_type=Fixed-point  arith_type=Unsigned  n_bits=1  bin_pt=0  preci_type=Single  exp_width=8  frac_width=24  explicit_period=off  period=1  equ=P=C  opselect=C  inp2=PCIN>>17  opr=+  inp1=P  carry=CIN  dbl_ovrd=off  block_type=constant
  Constant1 : xbsIndex_r4/Constant  const=lut_addr  gui_display_data_type=Fixed-point  arith_type=Unsigned  n_bits=4  bin_pt=0  preci_type=Single  exp_width=8  frac_width=24  explicit_period=off  period=1  equ=P=C  opselect=C  inp2=PCIN>>17  opr=+  inp1=P  carry=CIN  dbl_ovrd=off  block_type=constant
  Constant2 : xbsIndex_r4/Constant  const=0  gui_display_data_type=Fixed-point  arith_type=Unsigned  n_bits=1  bin_pt=0  preci_type=Single  exp_width=8  frac_width=24  explicit_period=off  period=1  equ=P=C  opselect=C  inp2=PCIN>>17  opr=+  inp1=P  carry=CIN  dbl_ovrd=off  block_type=constant
  Constant3 : xbsIndex_r4/Constant  const=band_sel  gui_display_data_type=Fixed-point  arith_type=Unsigned  n_bits=1  bin_pt=0  preci_type=Single  exp_width=8  frac_width=24  explicit_period=off  period=1  equ=P=C  opselect=C  inp2=PCIN>>17  opr=+  inp1=P  carry=CIN  dbl_ovrd=off  block_type=constant
  Constant4 : xbsIndex_r4/Constant  const=lut_addr  gui_display_data_type=Fixed-point  arith_type=Unsigned  n_bits=4  bin_pt=0  preci_type=Single  exp_width=8  frac_width=24  explicit_period=off  period=1  equ=P=C  opselect=C  inp2=PCIN>>17  opr=+  inp1=P  carry=CIN  dbl_ovrd=off  block_type=constant
  Constant5 : xbsIndex_r4/Constant  const=1  gui_display_data_type=Fixed-point  arith_type=Unsigned  n_bits=1  bin_pt=0  preci_type=Single  exp_width=8  frac_width=24  explicit_period=off  period=1  equ=P=C  opselect=C  inp2=PCIN>>17  opr=+  inp1=P  carry=CIN  dbl_ovrd=off  block_type=constant
  Convert : xbsIndex_r4/Convert  gui_display_data_type=Fixed-point  arith_type=Unsigned  n_bits=8  bin_pt=0  float_type=Single  exp_bits=8  fraction_bits=24  quantization=Truncate  overflow=Wrap  en=off  latency=0  pipeline=off  dbl_ovrd=off  block_type=convert
  Delay : xbsIndex_r4/Delay  rst=off  infoeditControl=Selection of Reset will increase slice count due to use of real FFs and instead of SRLs  en=off  latency=4  reg_retiming=off  dbl_ovrd=off  block_type=delay
      settings: infoedit=Hardware notes: A delay line is a chain, each link of which is an SRL16 or SRL32 followed by a flip-flop.
  Delay1 : xbsIndex_r4/Delay  rst=off  infoeditControl=Selection of Reset will increase slice count due to use of real FFs and instead of SRLs  en=off  latency=4  reg_retiming=off  dbl_ovrd=off  block_type=delay
      settings: infoedit=Hardware notes: A delay line is a chain, each link of which is an SRL16 or SRL32 followed by a flip-flop.
  Delay2 : xbsIndex_r4/Delay  rst=off  infoeditControl=Selection of Reset will increase slice count due to use of real FFs and instead of SRLs  en=off  latency=8  reg_retiming=off  dbl_ovrd=off  block_type=delay
      settings: infoedit=Hardware notes: A delay line is a chain, each link of which is an SRL16 or SRL32 followed by a flip-flop.
  Delay{3..6} (4 alike) : xbsIndex_r4/Delay  rst=off  infoeditControl=Selection of Reset will increase slice count due to use of real FFs and instead of SRLs  en=off  latency=1  reg_retiming=off  dbl_ovrd=off  block_type=delay
      settings: infoedit=Hardware notes: A delay line is a chain, each link of which is an SRL16 or SRL32 followed by a flip-flop.
  Reinterpret : xbsIndex_r4/Reinterpret  force_arith_type=on  arith_type="Signed  (2's comp)"  force_bin_pt=on  bin_pt=6  block_type=reinterpret
  addr1 : xbsIndex_r4/Concat  num_inputs=2  dbl_ovrd=off  block_type=concat
  addr3 : xbsIndex_r4/Concat  num_inputs=2  dbl_ovrd=off  block_type=concat
  addr_gen : Subsystem
  interp_a0 : Subsystem
  interp_a1 : Subsystem
  interp_b : Subsystem
  iqslice : Subsystem
  iqslice1 : Subsystem
  iqslice2 : Subsystem
  iqslice3 : Subsystem
  single_ram : lut_ram_vhdl/single_ram
  single_ram1 : lut_ram_vhdl/single_ram
  split_if1 : Subsystem
  split_if2 : Subsystem
  coef_iq : Outport
  wires:
  iqslice3/1(ciq) -> interp_a1/2(b1)
  iqslice2/1(ciq) -> interp_a1/1(b0)
  iqslice1/1(ciq) -> interp_a0/2(b1)
  Delay4/1 -> addr3/2
  Delay3/1 -> addr1/2
  Bus Selector1/6 -> single_ram1/10  "<active>"
  Bus Selector1/2 -> single_ram1/6  "<din>"
  Bus Selector1/7 -> single_ram1/11  "<per_clk>"
  Bus Selector1/1 -> single_ram1/5  "<addr>"
  Bus Selector1/5 -> single_ram1/9  "<bandsel >"
  Bus Selector1/4 -> single_ram1/8  "<chnsel>"
  Bus Selector1/3 -> single_ram1/7  "<we>"
  Constant5/1 -> single_ram1/4
  Constant4/1 -> single_ram1/2
  Constant3/1 -> single_ram1/3
  addr_gen/2(rd_addr1) -> single_ram1/1
  Bus Selector/1 -> single_ram/5  "<addr>"
  Bus Selector/2 -> single_ram/6  "<din>"
  Bus Selector/3 -> single_ram/7  "<we>"
  Bus Selector/4 -> single_ram/8  "<chnsel>"
  Bus Selector/5 -> single_ram/9  "<bandsel >"
  Bus Selector/6 -> single_ram/10  "<active>"
  Bus Selector/7 -> single_ram/11  "<per_clk>"
  per_wr/1 -> Bus Selector/1, Bus Selector1/1
  Constant2/1 -> single_ram/4
  Constant/1 -> single_ram/3
  Constant1/1 -> single_ram/2
  addr_gen/1(rd_addr0) -> single_ram/1
  addr3/1 -> addr_gen/5(addr1)
  addr1/1 -> addr_gen/4(addr0)
  active1/1 -> Delay6/1
  active0/1 -> Delay5/1
  chn_seq/1 -> addr_gen/1(chn)
  split_if2/1(iaddr) -> [A]
  split_if1/1(iaddr) -> Bf/1(iaddr), Bp1/1(d), B/1(d)
  a/1 -> split_if2/1(d)
  b/1 -> split_if1/1(d)
  interp_b/1(q) -> coef_iq/1
  single_ram/2 -> iqslice1/1(d32)  "c1"
  single_ram1/2 -> iqslice3/1(d32)  "c3"
  single_ram1/1 -> iqslice2/1(d32)  "c2"
  interp_a0/1(q) -> interp_b/1(b0)
  split_if1/2(faddr) -> Bf/2(delta)
  Bp1/1(q) -> [B_plus]
  B/1(q) -> [B]
  Bf/1(q) -> [Bf]
  [Af] -> Delay1/1
  [Af] -> Delay/1
  [Bf] -> Delay2/1
  [B_plus] -> addr1/1
  [A] -> Delay3/1
  [B] -> addr3/1
  [A] -> Delay4/1
  single_ram/1 -> iqslice/1(d32)
  Delay/1 -> interp_a1/3(delta)
  Delay1/1 -> interp_a0/3(delta)
  Delay2/1 -> interp_b/3(delta)
  iqslice/1(ciq) -> interp_a0/1(b0)
  Reinterpret/1 -> [Af]
  split_if2/2(faddr) -> Convert/1
  Delay5/1 -> addr_gen/2(active0)
  Delay6/1 -> addr_gen/3(active1)
  interp_a1/1(q) -> interp_b/2(b1)
  Convert/1 -> Reinterpret/1
